simulink library "Aero_Lib"  (Simulink 7.5)
settings: Solver=ode45  StartTime=0.0  StopTime=10.0  RelTol=1e-3
values from neighbouring files (symbols this model uses):
  AC = FASER_config    [UAV_config.m]    (also in UAV_modelconfig.mat = )
libraries: FASER_Aero_Lib x3, aerolibasang x1, aerolibadyn x1, simulink x1, Ultrastick_Aero_Lib x1
settings Model: Creator=austinmurch  LastModifiedBy=austinmurch

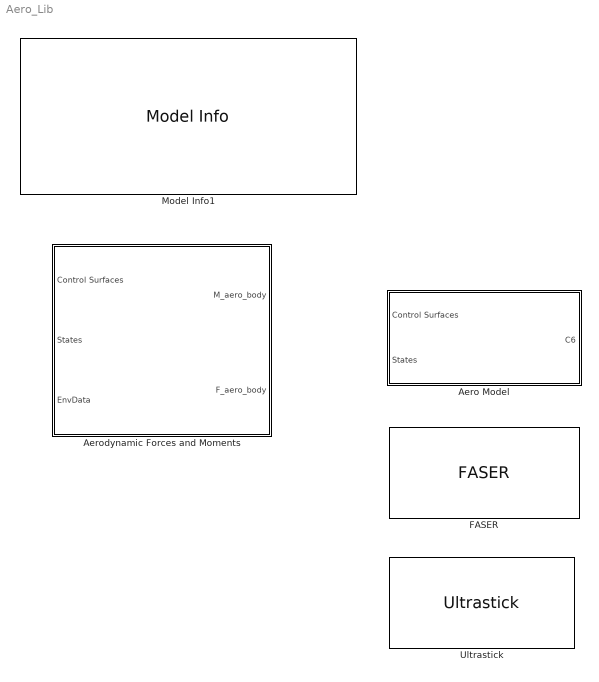
== system Aero_Lib ==
  Aero Model : Subsystem  BlockChoice=FASER
      settings: TemplateBlock=self  MemberBlocks=FASER,Ultrastick
  Aerodynamic Forces and Moments : Subsystem  mask{aeromodel=AC.Aero.use_FASER_aero}
      mask prompts: aeromodel "Aero Model Selection"
      mask help:
      | Set the boolean Aero Model Selection flag to 1 to use the FASER aerodynamic
      | model; otherwise, the Ultra Stick aero model will be used.
      |
      | This is done in this block's Mask Initialization commands. Also set is the
      | axes input for computing the forces and moments from the coefficients.
      mask init:
      | if aeromodel
      |     set_param([bdroot '/Nonlinear UAV Model/Forces and Moments/Aerodynamic Forces and Moments/Aero Model'],'BlockChoice','FASER')
      |     set_param([bdroot '/Nonlinear UAV Model/Forces and Moments/Aerodynamic Forces and Moments/Forces and Moments Calculation '],'inputAxes','Stability')
      |     set_param([bdroot '/Nonlinear UAV Model/Forces and Moments/Aerodynamic Forces and Moments/Forces and Moments Calculation '],'outputMomentAxes','Stability')
      | else
      |     set_param([bdroot '/Nonlinear UAV Model/Forces and Moments/Aerodynamic Forces and Moments/Aero Model'],'BlockChoice','Ultrastick')
      |     set_param([bdroot '/Nonlinear UAV Model/Forces and Moments/Aerodynamic Forces and Moments/Forces and Moments Calculation '],'inputAxes','Wind')
      |     set_param([bdroot '/Nonlinear UAV Model/Forces and Moments/Aerodynamic Forces and Moments/Forces and Moments Calculation '],'outputMomentAxes','Wind')
      | end
  FASER : FASER_Aero_Lib/FASER  SystemSampleTime=-1
  Model Info1 : simulink/Model-Wide Utilities/Model Info  SystemSampleTime=-1  InitialBlockCM=None  BlockCM=None  Frame=on  DisplayStringWithTags=|  HorizontalTextAlignment=Left  LeftAlignmentValue=0.02  SourceBlockDiagram=Aero_Lib  TagMaxNumber=20
      | MODEL INFORMATION
      | Aerodynamic Model Library
      | 
      | University of Minnesota
      | Aerospace Engineering and Mechanics
      | Copyright 2011 Regents of the University of Minnesota. All rights reserved.
      | 
      | == SVN Info ==
      | %<ModelVersion>
      | Last modified by %<LastModifiedBy> on %<LastModificationDate>
  Ultrastick : Ultrastick_Aero_Lib/Ultrastick  SystemSampleTime=-1

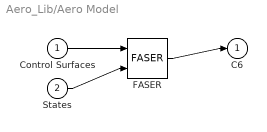
== system Aero_Lib/Aero Model ==
  Control Surfaces : Inport
  States : Inport  Port=2
  FASER : FASER_Aero_Lib/FASER  SystemSampleTime=-1
  C6 : Outport
  wires:
  Control Surfaces/1 -> FASER/1
  States/1 -> FASER/2
  FASER/1 -> C6/1

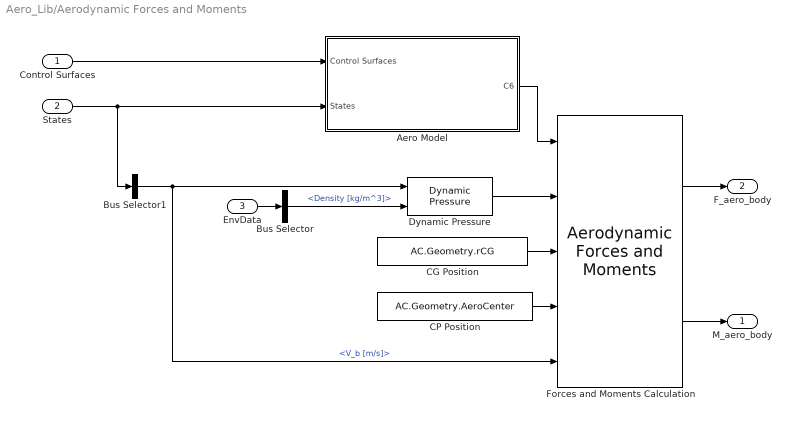
== system Aero_Lib/Aerodynamic Forces and Moments ==
  Control Surfaces : Inport  OutDataType=sfix(16)  OutScaling=2^0
  States : Inport  Port=2  OutDataType=sfix(16)  OutScaling=2^0
  EnvData : Inport  Port=3  OutDataType=sfix(16)  OutScaling=2^0
  Aero Model : Subsystem  BlockChoice=FASER
      settings: AttributesFormatString=%<BlockChoice>  TemplateBlock=Aero_Lib/Aero Model  MemberBlocks=FASER,Ultrastick
  Bus Selector : BusSelector  OutputSignals=Density [kg/m^3]
  Bus Selector1 : BusSelector  OutputSignals=V_b [m/s]
  CG Position : Constant  Value=AC.Geometry.rCG  OutDataType=sfix(16)  OutScaling=2^0
  CP Position : Constant  Value=AC.Geometry.AeroCenter  OutDataType=sfix(16)  OutScaling=2^0
  Dynamic Pressure : aerolibasang/Dynamic Pressure  SystemSampleTime=-1
  "Forces and Moments Calculation " : aerolibadyn/Aerodynamic Forces and Moments   SystemSampleTime=-1  inputAxes=Stability  outputForceAxes=Body  outputMomentAxes=Stability  S=AC.Geometry.S  b=AC.Geometry.b  cbar=AC.Geometry.c
  M_aero_body : Outport  OutDataType=sfix(16)  OutScaling=2^0
  F_aero_body : Outport  Port=2  OutDataType=sfix(16)  OutScaling=2^0
  wires:
  Bus Selector1/1 -> "Forces and Moments Calculation "/5, Dynamic Pressure/1  "<V_b [m/s]>"
  Aero Model/1(C6) -> "Forces and Moments Calculation "/1
  CG Position/1 -> "Forces and Moments Calculation "/3
  CP Position/1 -> "Forces and Moments Calculation "/4
  EnvData/1 -> Bus Selector/1
  States/1 -> Bus Selector1/1, Aero Model/2(States)
  Bus Selector/1 -> Dynamic Pressure/2  "<Density [kg/m^3]>"
  "Forces and Moments Calculation "/1 -> F_aero_body/1
  "Forces and Moments Calculation "/2 -> M_aero_body/1
  Dynamic Pressure/1 -> "Forces and Moments Calculation "/2
  Control Surfaces/1 -> Aero Model/1(Control Surfaces)

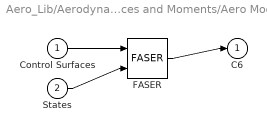
== system Aero_Lib/Aerodynamic Forces and Moments/Aero Model ==
  Control Surfaces : Inport
  States : Inport  Port=2
  FASER : FASER_Aero_Lib/FASER  SystemSampleTime=-1
  C6 : Outport
  wires:
  Control Surfaces/1 -> FASER/1
  States/1 -> FASER/2
  FASER/1 -> C6/1
